simulink model "motor_model"  (R2023a)
settings: Solver=VariableStepAuto  StartTime=0.0  StopTime=3  RelTol=1e-3
values from neighbouring files (symbols this model uses):
  J = (1/2) * motorMass * rotor_radius^2    (= 3.74e-05)    [motor_params.m]
  K_motor = 0.0136    [motor_params.m]
  R = 0.0830    (= 0.083)    [motor_params.m]
settings Model: Creator=Marcus  LastModifiedBy=Marcus

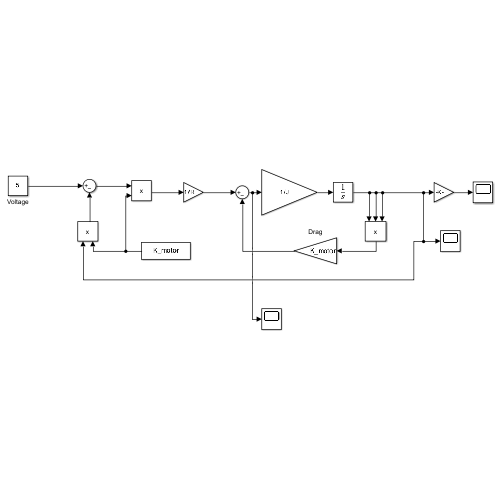
[thumbnail: Simulink's stored preview of the top-level diagram]
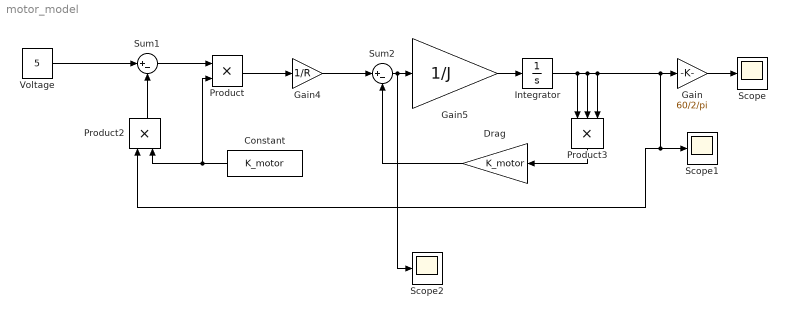
== system motor_model ==
  Constant : Constant  Value=K_motor
  Drag : Gain  Gain=K_motor
  Gain : Gain  Gain=60/2/pi
  Gain4 : Gain  Gain=1/R
  Gain5 : Gain  Gain=1/J
  Integrator : Integrator
  Product : Product
  Product2 : Product
  Product3 : Product  Inputs=3
  Scope : Scope
  Scope1 : Scope
  Scope2 : Scope
  Sum1 : Sum  Inputs=|+-
  Sum2 : Sum  Inputs=|+-
  Voltage : Constant  Value=5
  wires:
  Voltage/1 -> Sum1/1
  Product2/1 -> Sum1/2
  Sum1/1 -> Product/1
  Gain4/1 -> Sum2/1
  Product3/1 -> Drag/1
  Sum2/1 -> Scope2/1, Gain5/1
  Gain5/1 -> Integrator/1
  Integrator/1 -> Product3/3, Gain/1, Product2/1, Scope1/1, Product3/2, Product3/1
  Drag/1 -> Sum2/2
  Gain/1 -> Scope/1
  Product/1 -> Gain4/1
  Constant/1 -> Product2/2, Product/2
